simulink library "Window_Optics"  (R2018b)
settings: Solver=ode45  StartTime=0.0  StopTime=10.0  RelTol=1e-3  EnableMultiTasking=on
settings Model: Creator=lena.frank  LastModifiedBy=P41573
settings DataIOCC: LimitDataPoints=on  SaveFormat=Array  SignalLoggingSaveFormat=ModelDataLogs
settings OptimizationCC: ExpressionDepthLimit=2147483647  LifeSpan=inf
settings DebuggingCC: UnderspecifiedInitializationDetection=Classic  MergeDetectMultiDrivingBlocksExec=none  SolverPrmCheckMsg=warning  FcnCallInpInsideContextMsg=warning  StateNameClashWarn=warning  SFUnexpectedBacktrackingDiag=warning  SFNoUnconditionalDefaultTransitionDiag=warning  SFExecutionAtInitializationDiag=none
settings HardwareCC: ProdBitPerPointer=32  ProdBitPerSizeT=32  ProdBitPerPtrDiffT=32  ProdLargestAtomicFloat=None  ProdIntDivRoundTo=Undefined  ProdEndianess=Unspecified  ProdWordSize=32  ProdHWDeviceType=32-bit Generic
settings ModelReferenceCC: PropagateSignalLabelsOutOfModel=off
settings SFSimCC: SimUseLocalCustomCode=off
settings RTWCC: RTWUseLocalCustomCode=off
settings CodeAppCC: StateflowObjectComments=on
settings GRTTargetCC: TargetLangStandard=C89/C90 (ANSI)  GeneratePreprocessorConditionals=Disable all  CombineOutputUpdateFcns=off  GRTInterface=on
settings ConfigComp: CovMetricSettings=dw  CovHtmlReporting=on  CovSaveCumulativeToWorkspaceVar=on  CovSaveSingleToWorkspaceVar=on  CovExternalEMLEnable=off

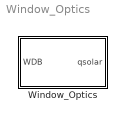
== system Window_Optics ==
  Window_Optics : Subsystem  mask(Window Optics){BreakpointsForDimension1=[-10 0 50 70 80 90], Table=[1.0 1.0  0.95  0.7  0.0  0.0], Gain=0.8}
      mask prompts: BreakpointsForDimension1 "Breakpoints for the incidence angle in degrees (0° = vertial)"; Table "Energetic transmission of direct sunlight at incidence angle breakpoints [0..1]"; Gain "Energetic light transmission for diffuse sunlight [0..1]"
      mask help: Light transission through the glasses. Data is a combination of glass properties (see taualfa.m) and geometry (shading).
      mask TypeOptions BreakpointsForDimension1: IAM window/BreakpointsForDimension1
      mask TypeOptions Table: IAM window/Table
      mask TypeOptions Gain: IAM diffuse/Gain

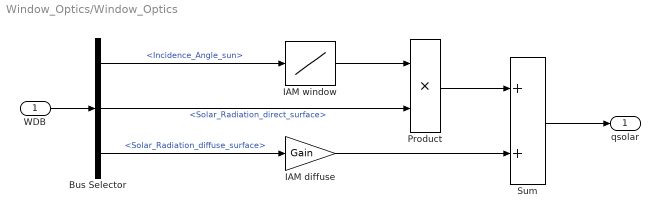
== system Window_Optics/Window_Optics ==
  WDB : Inport
  Bus Selector : BusSelector  OutputSignals=Incidence_Angle_sun,Solar_Radiation_direct_surface,Solar_Radiation_diffuse_surface
  IAM diffuse : Gain  Gain=Gain  SaturateOnIntegerOverflow=on  OutDataTypeStr=Inherit: Same as input  ParamDataTypeStr=Inherit: Same as input
  IAM window : Lookup_n-D  NumberOfTableDimensions=1  BreakpointsForDimension1=BreakpointsForDimension1  BeginIndexSearchUsingPreviousIndexResult=on  Table=Table  InternalRulePriority=Speed  RndMeth=Simplest  InputSameDT=on
  Product : Product
  Sum : Sum  SaturateOnIntegerOverflow=on  InputSameDT=on  OutDataTypeStr=Inherit: Same as first input
  qsolar : Outport
  wires:
  WDB/1 -> Bus Selector/1
  Bus Selector/2 -> Product/2  "<Solar_Radiation_direct_surface>"
  Bus Selector/1 -> IAM window/1  "<Incidence_Angle_sun>"
  Sum/1 -> qsolar/1
  Product/1 -> Sum/1
  IAM diffuse/1 -> Sum/2
  IAM window/1 -> Product/1
  Bus Selector/3 -> IAM diffuse/1  "<Solar_Radiation_diffuse_surface>"
